simulink model "Inverter Simulink file"  (R2023b)
settings: Solver=FixedStepAuto  StartTime=0.0  StopTime=5  RelTol=1e-3
libraries: spsMosfetLib x6, simulink x3, spsCurrentMeasurementLib x2, spsDCVoltageSourceLib x1, spsGroundLib x1, spsSeriesRLCBranchLib x1, spsThreePhaseSeriesRLCBranchLib x1, spsThreePhaseVIMeasurementLib x1, spsTriangleGeneratorLib x1, spsVoltageMeasurementLib x1, spspowerguiLib x1
settings Model: Creator=razwi  LastModifiedBy=razwi
settings DataIOCC: ReturnWorkspaceOutputs=off
settings RTWCC: GPUComputeCapability=5.0

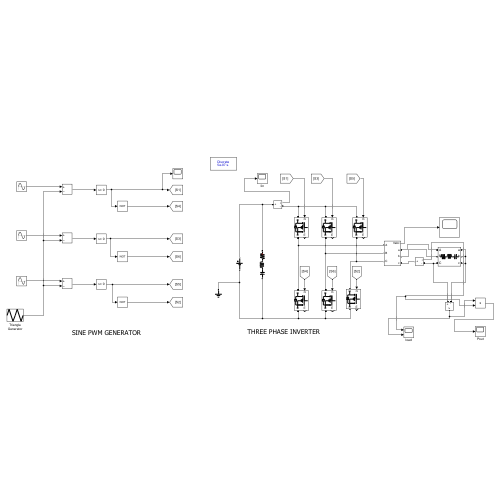
[thumbnail: Simulink's stored preview of the top-level diagram]
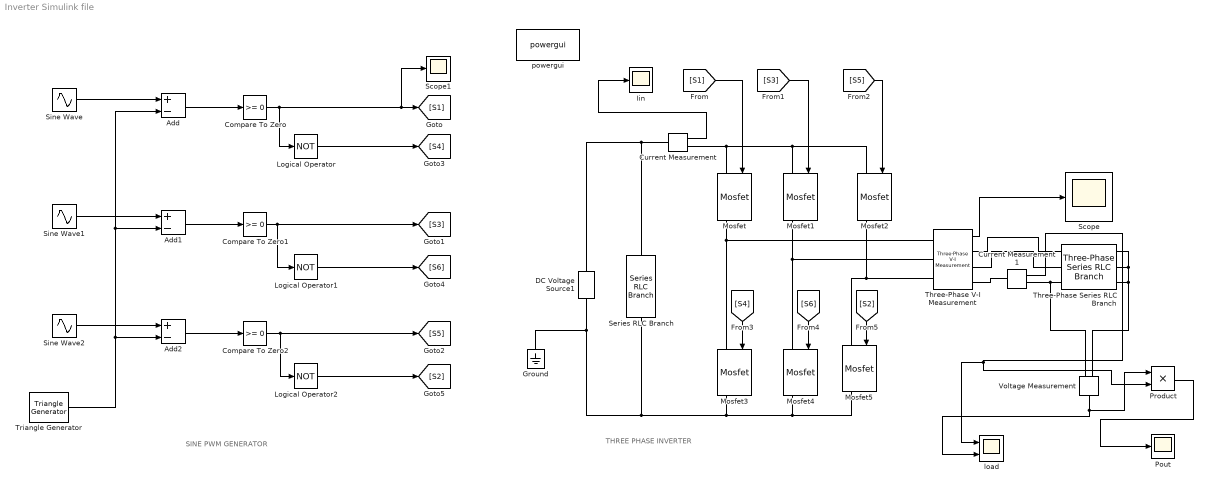
== system Inverter Simulink file ==
  note: SINE PWM GENERATOR
  note: THREE PHASE INVERTER
  Add : Sum  Inputs=+-
  Add1 : Sum  Inputs=+-
  Add2 : Sum  Inputs=+-
  Compare To Zero : simulink/Logic and Bit Operations/Compare To Zero  relop=>=  OutDataTypeStr=boolean
  Compare To Zero1 : simulink/Logic and Bit Operations/Compare To Zero  relop=>=  OutDataTypeStr=boolean
  Compare To Zero2 : simulink/Logic and Bit Operations/Compare To Zero  relop=>=  OutDataTypeStr=boolean
  Current Measurement : spsCurrentMeasurementLib/Current Measurement  PhasorSimulation=off  OutputType=Complex  PSBequivalent=0
  Current Measurement1 : spsCurrentMeasurementLib/Current Measurement  PhasorSimulation=off  OutputType=Complex  PSBequivalent=0
  DC Voltage Source1 : spsDCVoltageSourceLib/DC Voltage Source  Amplitude=540  Measurements=None
  Ground : spsGroundLib/Ground  LConnTagsString=a
  Iin : Scope
  Logical Operator : Logic  Operator=NOT  AllPortsSameDT=off  OutDataTypeStr=boolean
  Logical Operator1 : Logic  Operator=NOT  AllPortsSameDT=off  OutDataTypeStr=boolean
  Logical Operator2 : Logic  Operator=NOT  AllPortsSameDT=off  OutDataTypeStr=boolean
  Mosfet{,1..5} (6 alike) : spsMosfetLib/Mosfet  Ron=0.039  Lon=0  Rd=0.093  Vfd=4  IC=0  Rs=5e4  Cs=inf  Measurements=on
  Pout : Scope
  Product : Product
  Scope : Scope
  Scope1 : Scope
  Series RLC Branch : spsSeriesRLCBranchLib/Series RLC Branch  LConnTagsString=__new0  RConnTagsString=__new0  BranchType=RLC  Resistance=0.1  Inductance=0  SetiL0=off  InitialCurrent=0  Capacitance=1e-5  Setx0=off  InitialVoltage=0  Measurements=None
  Sine Wave : Sin  Amplitude=0.8  Frequency=50*2*pi  SampleTime=0
  Sine Wave1 : Sin  Amplitude=0.8  Frequency=50*2*pi  Phase=2*pi/3  SampleTime=0
  Sine Wave2 : Sin  Amplitude=0.8  Frequency=50*2*pi  Phase=4*pi/3  SampleTime=0
  Three-Phase Series RLC Branch : spsThreePhaseSeriesRLCBranchLib/Three-Phase Series RLC Branch  LConnTagsString=A|B|C  RConnTagsString=A|B|C  BranchType=RLC  Resistance=10  Inductance=20e-3  Capacitance=0  Measurements=None
  Three-Phase V-I Measurement : spsThreePhaseVIMeasurementLib/Three-Phase V-I Measurement  VoltageMeasurement=phase-to-ground  SetLabelV=off  LabelV=Vabc  Vpu=off  VpuLL=off  CurrentMeasurement=no  SetLabelI=off  LabelI=Iabc  Ipu=off  Pbase=100e6  Vbase=500e3  OutputType=Complex  PhasorSimulation=off  PSBequivalent=0
  Triangle Generator : spsTriangleGeneratorLib/Triangle Generator  Freq=10000  Phase=90  Ts=0
  Voltage Measurement : spsVoltageMeasurementLib/Voltage Measurement  PhasorSimulation=off  OutputType=Complex  PSBequivalent=0
  load : Scope  NumInputPorts=2
  powergui : spspowerguiLib/powergui  Priority=1  SimulationMode=Discrete  SampleTime=5e-7  frequency=60  Iterations=50  frequencyindice=0  Pbase=100e6  ErrMax=1e-4  UnitsV=kV  UnitsW=MW  buscounter=0  FunctionMessages=off  echomessages=off  EnableUseOfTLC=off  CurrentSourceSwitches=off  DisableSnubberDevices=off  DisableRonSwitches=off  DisableVfSwitches=off  DisplayEquations=off  AutomaticDiscreteSolvers=off  SolverType=Tustin/Backward Euler (TBE)  Interpol=off  ExternalGateDelay=off  methode=off  Ts=100  x0status=blocks  SPID=on  SwTol=0  HookPort=off  NonlinearTolerance=1e-4  nMaxIteration=100  ContinueOnMaxIteration=off  RestoreLinks=warning  ResistiveCurrentMeasurement=off  Frange=[0:2:500]  Ylog=off  Xlog=on  ShowGrid=off  save=off  variable=ZData  structure=0  ZoomFFT=off  StartTime=0.0  cycles=1  DisplayStyle=1  fundamental=60  FreqAxis=off  MaxFrequency=1000  frequencyindicesteady=1  RmsSteady=1  display=off
  wires:
  Add/1 -> Compare To Zero/1
  Add2/1 -> Compare To Zero2/1
  Logical Operator1/1 -> [S6]
  Compare To Zero/1 -> Scope1/1, [S1], Logical Operator/1
  Compare To Zero2/1 -> [S5], Logical Operator2/1
  Triangle Generator/1 -> Add/2, Add1/2, Add2/2
  Compare To Zero1/1 -> [S3], Logical Operator1/1
  Sine Wave/1 -> Add/1
  Sine Wave1/1 -> Add1/1
  Add1/1 -> Compare To Zero1/1
  Sine Wave2/1 -> Add2/1
  Voltage Measurement/1 -> Product/1, load/2
  Three-Phase V-I Measurement/1 -> Scope/1
  [S3] -> Mosfet1/1
  [S1] -> Mosfet/1
  [S2] -> Mosfet5/1
  [S5] -> Mosfet2/1
  Current Measurement/1 -> Iin/1
  Current Measurement1/1 -> Product/2, load/1
  Product/1 -> Pout/1
  [S4] -> Mosfet3/1
  [S6] -> Mosfet4/1
  Logical Operator/1 -> [S4]
  Logical Operator2/1 -> [S2]
  connections:
  Three-Phase Series RLC Branch/RConn3 -- Three-Phase Series RLC Branch/RConn1 -- Three-Phase Series RLC Branch/RConn2 -- Voltage Measurement/LConn2
  Current Measurement1/RConn1 -- Voltage Measurement/LConn1 -- Three-Phase Series RLC Branch/LConn3
  Mosfet3/RConn1 -- Series RLC Branch/RConn1 -- DC Voltage Source1/LConn1 -- Ground/LConn1 -- Mosfet5/RConn1 -- Mosfet4/RConn1
  Mosfet/RConn1 -- Mosfet3/LConn1 -- Three-Phase V-I Measurement/LConn1
  Three-Phase V-I Measurement/LConn2 -- Mosfet4/LConn1 -- Mosfet1/RConn1
  Mosfet/LConn1 -- Mosfet2/LConn1 -- Mosfet1/LConn1 -- Current Measurement/RConn1
  Three-Phase V-I Measurement/LConn3 -- Mosfet5/LConn1 -- Mosfet2/RConn1
  Three-Phase V-I Measurement/RConn3 -- Current Measurement1/LConn1
  DC Voltage Source1/RConn1 -- Series RLC Branch/LConn1 -- Current Measurement/LConn1
  Three-Phase V-I Measurement/RConn2 -- Three-Phase Series RLC Branch/LConn2
  Three-Phase V-I Measurement/RConn1 -- Three-Phase Series RLC Branch/LConn1
